simulink model "simulinkSimulacion"  (R2018b)
settings: Solver=FixedStepAuto  StartTime=0.0  StopTime=10  FixedStep=0.005  RelTol=1e-3
undefined symbols (not defined in the file): AHat, BHat, CHat, DHat, EEd, EEdObs, FHat, K, kgainObs
settings Model: Creator=a4lfr  LastModifiedBy=AlfredoMaussa

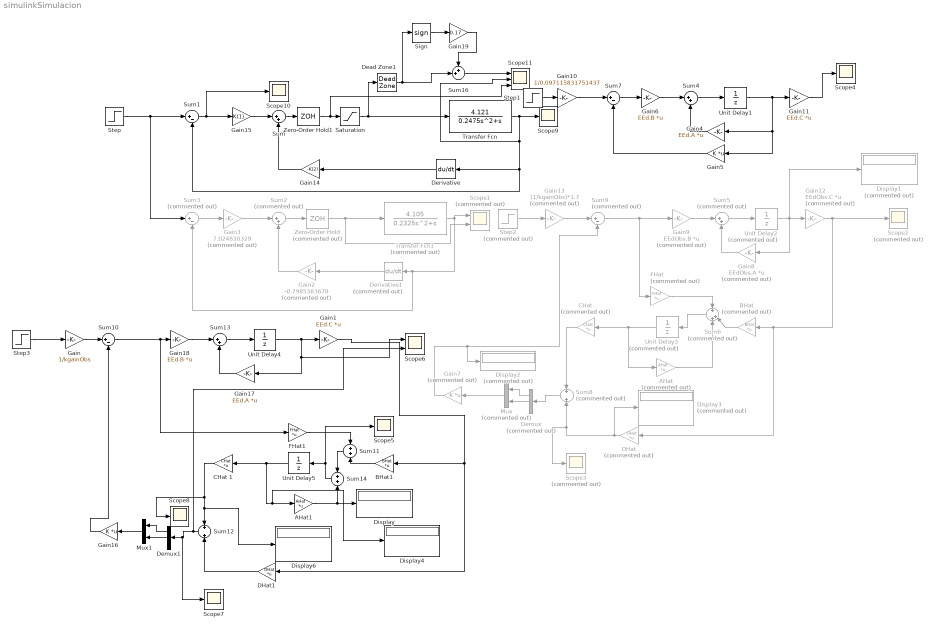
== system simulinkSimulacion ==
  AHat : Gain  Commented=on  Gain=AHat  Multiplication=Matrix(K*u)
  AHat1 : Gain  Gain=AHat  Multiplication=Matrix(K*u)
  BHat : Gain  Commented=on  Gain=BHat  Multiplication=Matrix(K*u)
  BHat1 : Gain  Gain=BHat  Multiplication=Matrix(K*u)
  "CHat " : Gain  Commented=on  Gain=CHat  Multiplication=Matrix(K*u)
  CHat 1 : Gain  Gain=CHat  Multiplication=Matrix(K*u)
  DHat : Gain  Commented=on  Gain=DHat  Multiplication=Matrix(K*u)
  DHat1 : Gain  Gain=DHat  Multiplication=Matrix(K*u)
  Dead Zone1 : DeadZone  LowerValue=-0.17  UpperValue=0.17  SaturateOnIntegerOverflow=on
  Demux : Demux  Commented=on  Outputs=3
  Demux1 : Demux  Outputs=3
  Derivative : Derivative  CoefficientInTFapproximation=100
  Derivative1 : Derivative  Commented=on  CoefficientInTFapproximation=100
  Display : Display
  Display1 : Display  Commented=on
  Display2 : Display  Commented=on
  Display3 : Display  Commented=on
  Display4 : Display
  Display6 : Display
  FHat : Gain  Commented=on  Gain=FHat  Multiplication=Matrix(K*u)
  FHat1 : Gain  Gain=FHat  Multiplication=Matrix(K*u)
  Gain : Gain  Gain=1/kgainObs
  Gain1 : Gain  Gain=EEd.C  Multiplication=Matrix(K*u)
  Gain10 : Gain  Gain=1/0.097115831751437
  Gain11 : Gain  Gain=EEd.C  Multiplication=Matrix(K*u)
  Gain12 : Gain  Commented=on  Gain=EEdObs.C  Multiplication=Matrix(K*u)
  Gain13 : Gain  Commented=on  Gain=(1/kgainObs)*1.7
  Gain14 : Gain  Gain=-K(2)
  Gain15 : Gain  Gain=K(1)
  Gain16 : Gain  Gain=K  Multiplication=Matrix(K*u)
  Gain17 : Gain  Gain=EEd.A  Multiplication=Matrix(K*u)
  Gain18 : Gain  Gain=EEd.B  Multiplication=Matrix(K*u)
  Gain19 : Gain  Gain=0.17
  Gain2 : Gain  Commented=on  Gain=-0.7985383678
  Gain3 : Gain  Commented=on  Gain=7.024830329
  Gain4 : Gain  Gain=EEd.A  Multiplication=Matrix(K*u)
  Gain5 : Gain  Gain=K  Multiplication=Matrix(K*u)
  Gain6 : Gain  Gain=EEd.B  Multiplication=Matrix(K*u)
  Gain7 : Gain  Commented=on  Gain=K  Multiplication=Matrix(K*u)
  Gain8 : Gain  Commented=on  Gain=EEdObs.A  Multiplication=Matrix(K*u)
  Gain9 : Gain  Commented=on  Gain=EEdObs.B  Multiplication=Matrix(K*u)
  Mux : Mux  Commented=on  Inputs=2
  Mux1 : Mux  Inputs=2
  Saturation : Saturate  UpperLimit=1  LowerLimit=-1
  Scope1 : Scope  Commented=on  NumInputPorts=2
  Scope{4..5,7..10} (6 alike) : Scope
  Scope11 : Scope  NumInputPorts=3
  Scope2 : Scope  Commented=on
  Scope3 : Scope  Commented=on
  Scope6 : Scope  NumInputPorts=2
  Sign : Signum
  Step : Step  Time=0  SampleTime=0
  Step1 : Step  Time=0  SampleTime=0
  Step2 : Step  Commented=on  Time=0  SampleTime=0
  Step3 : Step  Time=0  SampleTime=0
  Sum : Sum  Inputs=|++
  Sum1 : Sum  Inputs=|+-
  Sum10 : Sum  Inputs=|+-
  Sum11 : Sum  Inputs=+|+
  Sum12 : Sum  Inputs=+||+
  Sum13 : Sum  Inputs=|++
  Sum14 : Sum  Inputs=+|+
  Sum16 : Sum  Inputs=++|
  Sum2 : Sum  Commented=on  Inputs=|++
  Sum3 : Sum  Commented=on  Inputs=|+-
  Sum4 : Sum  Inputs=|++
  Sum5 : Sum  Commented=on  Inputs=|++
  Sum6 : Sum  Commented=on  Inputs=+|++
  Sum7 : Sum  Inputs=|+-
  Sum8 : Sum  Commented=on  Inputs=+||+
  Sum9 : Sum  Commented=on  Inputs=|+-
  Transfer Fcn : TransferFcn  Numerator=[4.121]  Denominator=[0.2475 1 0]
  Transfer Fcn1 : TransferFcn  Commented=on  Numerator=[4.105]  Denominator=[0.2325 1 0]
  Unit Delay1 : UnitDelay  SampleTime=0.005
  Unit Delay2 : UnitDelay  Commented=on  InitialCondition=[0,0,30]  SampleTime=0.005
  Unit Delay3 : UnitDelay  Commented=on  SampleTime=0.005
  Unit Delay4 : UnitDelay  SampleTime=0.005
  Unit Delay5 : UnitDelay  InitialCondition=[0,0]  SampleTime=0.005
  Zero-Order Hold : ZeroOrderHold  Commented=on  SampleTime=0.005
  Zero-Order Hold1 : ZeroOrderHold  SampleTime=0.005
  wires:
  Transfer Fcn/1 -> Scope11/2, Derivative/1, Sum1/2, Scope9/1
  Derivative/1 -> Gain14/1
  Gain14/1 -> Sum/2
  Sum1/1 -> Scope10/1, Gain15/1
  Gain15/1 -> Sum/1
  Gain3/1 -> Sum2/1
  Sum3/1 -> Gain3/1
  Step/1 -> Sum3/1, Sum1/1
  Gain2/1 -> Sum2/2
  Derivative1/1 -> Gain2/1
  Transfer Fcn1/1 -> Scope1/1, Sum3/2, Derivative1/1
  Sum2/1 -> Zero-Order Hold/1
  Zero-Order Hold/1 -> Scope1/2, Transfer Fcn1/1
  Sum/1 -> Zero-Order Hold1/1
  Zero-Order Hold1/1 -> Scope11/3, Saturation/1
  Sum4/1 -> Unit Delay1/1
  Gain4/1 -> Sum4/2
  Gain6/1 -> Sum4/1
  Sum7/1 -> Gain6/1
  Gain5/1 -> Sum7/2
  Step1/1 -> Gain10/1
  Gain10/1 -> Sum7/1
  Unit Delay1/1 -> Gain11/1, Gain5/1, Gain4/1
  Unit Delay2/1 -> Gain8/1, Display1/1, Gain12/1
  Gain9/1 -> Sum5/1
  Gain8/1 -> Sum5/2
  Sum5/1 -> Unit Delay2/1
  FHat/1 -> Sum6/1
  BHat/1 -> Sum6/2
  Sum6/1 -> Unit Delay3/1
  Unit Delay3/1 -> AHat/1, "CHat "/1
  "CHat "/1 -> Sum8/1
  DHat/1 -> Display3/1, Sum8/2, Scope3/1
  Gain12/1 -> DHat/1, BHat/1, Scope2/1
  AHat/1 -> Sum6/3
  Sum9/1 -> FHat/1, Gain9/1
  Gain7/1 -> Display2/1, Sum9/2
  Demux/1 -> Mux/1
  Demux/2 -> Mux/2
  Mux/1 -> Gain7/1
  Gain11/1 -> Scope4/1
  Step2/1 -> Gain13/1
  Gain13/1 -> Sum9/1
  Sum8/1 -> Demux/1
  Sum12/1 -> Scope6/2, Scope7/1, Demux1/1
  Mux1/1 -> Gain16/1
  Demux1/2 -> Mux1/2
  Demux1/1 -> Mux1/1
  Gain1/1 -> DHat1/1, BHat1/1
  DHat1/1 -> Sum12/2
  CHat 1/1 -> Sum12/1, Display6/1, Scope8/1
  Unit Delay5/1 -> CHat 1/1, Display4/1, AHat1/1
  BHat1/1 -> Sum11/2
  FHat1/1 -> Sum11/1
  Sum11/1 -> Sum14/1
  Sum14/1 -> Scope5/1, Unit Delay5/1
  AHat1/1 -> Sum14/2, Display/1
  Unit Delay4/1 -> Scope6/1, Gain17/1, Gain1/1
  Sum10/1 -> FHat1/1, Gain18/1
  Gain18/1 -> Sum13/1
  Gain17/1 -> Sum13/2
  Sum13/1 -> Unit Delay4/1
  Gain16/1 -> Sum10/2
  Step3/1 -> Gain/1
  Gain/1 -> Sum10/1
  Dead Zone1/1 -> Sign/1, Sum16/2
  Sign/1 -> Gain19/1
  Gain19/1 -> Sum16/1
  Saturation/1 -> Transfer Fcn/1, Dead Zone1/1
  Sum16/1 -> Scope11/1
